simulink model "Octocopter2D"  (R2017b)
settings: Solver=VariableStepAuto  StartTime=0.0  StopTime=10  MaxStep=1e-3  RelTol=1e-3
undefined symbols (not defined in the file): Initial
libraries: simulink_extras x2
settings Model: Creator=jeremie  LastModifiedBy=jeremie

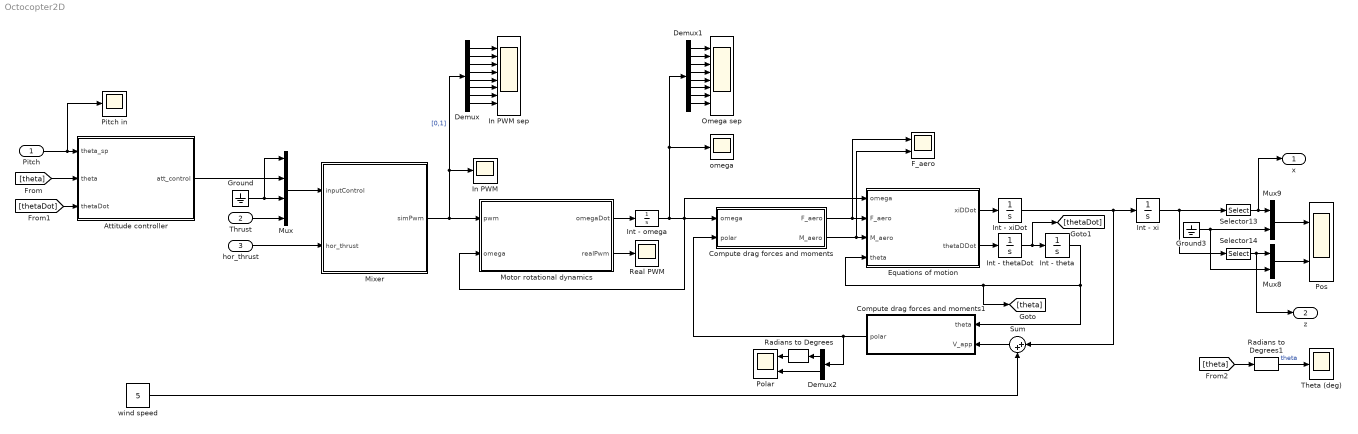
== system Octocopter2D ==
  Pitch : Inport
  Thrust : Inport  Port=2
  hor_thrust : Inport  Port=3
  Attitude controller : Subsystem
  Compute drag forces and moments : MATLAB Function  TreatAsAtomicUnit=on
  Compute drag forces and moments1 : MATLAB Function  TreatAsAtomicUnit=on
  Demux : Demux  Outputs=8
  Demux1 : Demux  Outputs=8
  Demux2 : Demux  Outputs=2
  Equations of motion : MATLAB Function  TreatAsAtomicUnit=on
  F_aero : Scope  NumInputPorts=2
  Ground : Ground
  Ground3 : Ground
  In PWM : Scope
  In PWM sep : Scope  NumInputPorts=8
  Int - omega : Integrator  InitialCondition=Initial.OMEGA
  Int - theta : Integrator
  Int - thetaDot : Integrator
  Int - xi : Integrator
  Int - xiDot : Integrator
  Mixer : MATLAB Function  TreatAsAtomicUnit=on
  Motor rotational dynamics : MATLAB Function  TreatAsAtomicUnit=on
  Mux : Mux
  Mux8 : Mux  Inputs=2
  Mux9 : Mux  Inputs=2
  Omega sep : Scope  NumInputPorts=8
  Pitch in : Scope
  Polar : Scope  NumInputPorts=2
  Pos : Scope  NumInputPorts=2
  Radians to Degrees : simulink_extras/Transformations/Radians to Degrees
  Radians to Degrees1 : simulink_extras/Transformations/Radians to Degrees
  Real PWM : Scope
  Selector13 : Selector  InputPortWidth=2  IndexOptions=Index vector (dialog)  Indices=1  OutputSizes=1
  Selector14 : Selector  InputPortWidth=2  IndexOptions=Index vector (dialog)  Indices=2  OutputSizes=1
  Sum : Sum  Inputs=|++
  Theta (deg) : Scope
  omega : Scope
  wind speed : Constant  Value=5
  x : Outport
  z : Outport  Port=2
  wires:
  Int - omega/1 -> Equations of motion/1(omega), Compute drag forces and moments/1(omega), Motor rotational dynamics/2(omega), omega/1, Demux1/1
  Compute drag forces and moments/1(F_aero) -> F_aero/1, Equations of motion/2(F_aero)
  Compute drag forces and moments/2(M_aero) -> F_aero/2, Equations of motion/3(M_aero)
  Motor rotational dynamics/1(omegaDot) -> Int - omega/1
  Motor rotational dynamics/2(realPwm) -> Real PWM/1
  Mixer/1(simPwm) -> Motor rotational dynamics/1(pwm), Demux/1, In PWM/1  "[0,1]"
  Mux/1 -> Mixer/1(inputControl)
  Ground/1 -> Mux/3, Mux/1
  Attitude controller/1(att_control) -> Mux/2
  Thrust/1 -> Mux/4
  Equations of motion/1(xiDDot) -> Int - xiDot/1
  Int - xiDot/1 -> Sum/1, Int - xi/1
  Equations of motion/2(thetaDDot) -> Int - thetaDot/1
  Int - thetaDot/1 -> [thetaDot], Int - theta/1
  Int - theta/1 -> [theta], Equations of motion/4(theta), Compute drag forces and moments1/1(theta)
  wind speed/1 -> Sum/2
  Sum/1 -> Compute drag forces and moments1/2(V_app)
  Compute drag forces and moments1/1(polar) -> Demux2/1, Compute drag forces and moments/2(polar)
  Ground3/1 -> Mux8/2, Mux9/2
  Selector14/1 -> z/1, Mux8/1
  Selector13/1 -> x/1, Mux9/1
  Mux8/1 -> Pos/2
  Mux9/1 -> Pos/1
  Int - xi/1 -> Selector14/1, Selector13/1
  Demux/1 -> In PWM sep/1
  Demux/2 -> In PWM sep/2
  Demux/3 -> In PWM sep/3
  Demux/4 -> In PWM sep/4
  Demux/5 -> In PWM sep/5
  Demux/6 -> In PWM sep/6
  Demux/7 -> In PWM sep/7
  Demux/8 -> In PWM sep/8
  Demux1/8 -> Omega sep/8
  Demux1/7 -> Omega sep/7
  Demux1/6 -> Omega sep/6
  Demux1/5 -> Omega sep/5
  Demux1/4 -> Omega sep/4
  Demux1/3 -> Omega sep/3
  Demux1/2 -> Omega sep/2
  Demux1/1 -> Omega sep/1
  Demux2/2 -> Polar/2
  Demux2/1 -> Radians to Degrees/1
  Radians to Degrees/1 -> Polar/1
  Radians to Degrees1/1 -> Theta (deg)/1  "theta"
  Pitch/1 -> Pitch in/1, Attitude controller/1(theta_sp)
  [theta] -> Attitude controller/2(theta)
  [thetaDot] -> Attitude controller/3(thetaDot)
  hor_thrust/1 -> Mixer/2(hor_thrust)
  [theta] -> Radians to Degrees1/1

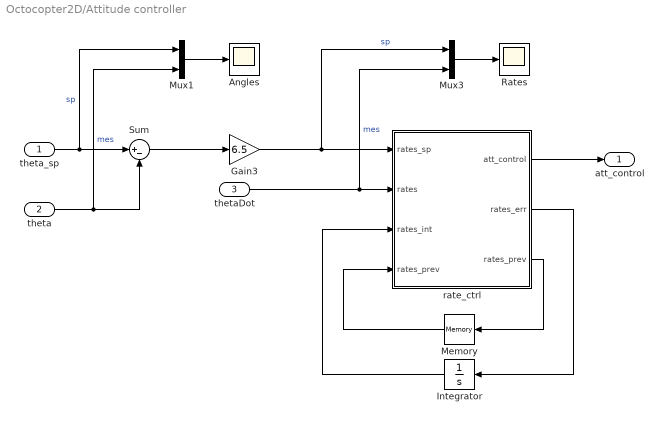
== system Octocopter2D/Attitude controller ==
  theta_sp : Inport
  theta : Inport  Port=2
  thetaDot : Inport  Port=3
  Angles : Scope
  Gain3 : Gain  Gain=6.5
  Integrator : Integrator
  Memory : Memory
  Mux1 : Mux  Inputs=2
  Mux3 : Mux  Inputs=2
  Rates : Scope
  Sum : Sum  Inputs=|+-
  rate_ctrl : MATLAB Function  TreatAsAtomicUnit=on  SystemSampleTime=0.002
  att_control : Outport
  wires:
  rate_ctrl/2(rates_err) -> Integrator/1
  rate_ctrl/3(rates_prev) -> Memory/1
  Integrator/1 -> rate_ctrl/3(rates_int)
  rate_ctrl/1(att_control) -> att_control/1
  Memory/1 -> rate_ctrl/4("rates_prev ")
  Mux3/1 -> Rates/1
  thetaDot/1 -> rate_ctrl/2(rates), Mux3/2  "mes"
  Gain3/1 -> rate_ctrl/1(rates_sp), Mux3/1  "sp"
  Sum/1 -> Gain3/1
  theta_sp/1 -> Mux1/1, Sum/1  "sp"
  theta/1 -> Mux1/2, Sum/2  "mes"
  Mux1/1 -> Angles/1

== matlab function Octocopter2D/Attitude controller/rate_ctrl ==
  data: rates_sp input size=1; rates input size=1; att_control output size=1; rates_err output; rates_prev output; rates_int input size=1; rates_prev input size=1
function [ att_control, rates_err, rates_prev ] = rate_ctrl(rates_sp, rates, rates_int, rates_prev)
rates_p = 0.15;
rates_i = 0.05;
rates_d = 0.003;
rate_ff = 0;

dt = 0.002;

% Angular rates error
rates_err = - rates_sp + rates;

% % Perform the integration using a first order method and do not propaate the result if out of range or invalid
% rates_int = rates_int +  rates_err * dt;

att_control = rates_p .* rates_err + rates_i .* rates_int + rates_d .* (rates_prev - rates) ./ dt + rate_ff .* rates_sp;

rates_prev = rates;

end

== matlab function Octocopter2D/Compute drag forces and moments ==
  data: omega input; polar input size=2; F_aero output; M_aero output; Uav parameter
function [F_aero, M_aero] = computeAero( omega, polar, Uav )
%#codegen

% Name variables
alpha    = -polar(1); % equations assume alpha measured the other way
U        = polar(2);
omegaBar = mean(omega);
rho      = Uav.RHO_AIR;
D_UAV    = Uav.D_UAV;
A_UAV    = Uav.A_UAV;
D_PROP   = Uav.D_PROP;
A_PROP   = Uav.A_PROP;
n        = Uav.N_ROTORS;

% Force coefficients
Cxb1 = -0.241*cos(alpha) + 0.036*cos(3*alpha) + 0.016*cos(7*alpha);
Cxb2 = -0.053*cos(alpha) - 0.008*cos(3*alpha);
Czb1 = -0.724*sin(alpha) + 0.080;
Czb2 = -0.222*sin(alpha) + 0.065;

% Moment coefficients
lambda = omegaBar*D_PROP / ( 2*U );
A1  =  0.116 * ( 1 - exp(-0.126*lambda) );
A2  = -0.041 * ( 1 - exp(-0.308*lambda) );
CM1 =  0.009*cos(alpha) + 0.003*cos(3*alpha) - 0.014*sin(2*alpha);
CM2 =  A1*cos(alpha) + A2*sin(2*alpha);

% Forces and moments
Fxb = 0.5*rho*U^2*Cxb1*A_UAV      + 0.5*rho*U*omegaBar*Cxb2*D_PROP*A_PROP*(n/4);
Fzb = 0.5*rho*U^2*Czb1*A_UAV      + 0.5*rho*U*omegaBar*Czb2*D_PROP*A_PROP*(n/4);
M   = 0.5*rho*U^2*CM1*A_UAV*D_UAV + 0.5*rho*U*omegaBar*CM2*D_PROP^2*A_PROP*(n/4);

% Output forces - NED
F_aero = [ Fxb; -Fzb ];
M_aero = M;

== matlab function Octocopter2D/Motor rotational dynamics ==
  data: pwm input; omegaDot output; omega input; realPwm output
function [omegaDot, realPwm]  = motorRotDynamics( pwm, omega)
%#codegen

realPwm = (1000 * pwm + 1000);
rotorTimeConst = 7.006512e-02;
omegaRef = zeros(8,1);
omegaRef = 0.84*(7.969173e-1 .* realPwm - 6.528579e2);

omegaDot = (omegaRef - omega) / rotorTimeConst;

== matlab function Octocopter2D/Equations of motion ==
  data: omega input; xiDDot output; F_aero input; M_aero input; theta input; thetaDDot output; Uav parameter
function [ xiDDot, thetaDDot ] = Octo2DModel( omega, F_aero, M_aero, theta, Uav )
%#codegen

% Name variables
m_UAV = Uav.M;
J_UAV = Uav.J;
C_T   = Uav.C_T;
D_UAV = Uav.D_UAV;
Fxb = F_aero(1);
Fzb = F_aero(2);
g = 9.80665;
zeta = Uav.ZETA;

% Forces and pitching moment in body frame
T   = -cos(zeta)*C_T*sum(omega.^2);
Txb = 2*sin(zeta)*C_T*(omega(3)^2 - omega(2)^2);

M = 2*cos(zeta)*D_UAV*C_T * ( ...
    omega(1)^2*sind(22.5) + omega(2)^2*cosd(22.5) - ...
    omega(3)^2*cosd(22.5) - omega(4)^2*sind(22.5) );

% Forces and pitching moment in world frame
xDDot = ( (T + Fzb)*sin(theta) + (Txb + Fxb)*cos(theta) ) / m_UAV;
zDDot = ( (T + Fzb)*cos(theta) + (Txb + Fxb)*sin(theta) + m_UAV*g ) / m_UAV;

xiDDot = [xDDot; zDDot];
thetaDDot = (M + M_aero) / J_UAV;

end

== matlab function Octocopter2D/Mixer ==
  data: inputControl input size=4; simPwm output size=8; hor_thrust input
function simPwm = mix( inputControl, hor_thrust )
%#codegen
    ROTOR_COUNT = 8;
    a = tand(22.5);
    rotors = struct( 'roll_scale',   {-0.095671,  0.095671, -0.230970, -0.095671,  0.095671,  0.230970,  0.230970, -0.230970}, ...
                     'pitch_scale',  { 0.230970, -0.230970,  0.095671, -0.230970,  0.230970, -0.095671,  0.095671, -0.095671}, ...
                     'yaw_scale',    {-2.500000, -2.500000,  2.500000,  2.500000,  2.500000,  2.500000, -2.500000, -2.500000}, ...
                     'thrust_scale', { 0.125000,  0.125000,  0.125000,  0.125000,  0.125000,  0.125000,  0.125000,  0.125000}, ...
                     'hor_thrust_scale', { a*1,  -a*1,  -1,  -a*1,  a*1,  1,  -1,  1});

%     roll   = constrain(inputControl(1), -1.0, 1.0);
%     pitch  = constrain(inputControl(2), -1.0, 1.0);
%     yaw    = constrain(inputControl(3), -1.0, 1.0);
%     thrust = constrain(inputControl(4), 0.0, 1.0);
%     min_out = 0.0;
%     max_out = 0.0;
%

    roll   = inputControl(1);
    pitch  = -inputControl(2);
    yaw    = -inputControl(3);
    thrust = inputControl(4);
    outputControl = zeros(ROTOR_COUNT,1);

    % /* perform initial mix pass yielding unbounded outputs, ignore yaw */
    for i = 1:ROTOR_COUNT
        out = pitch * rotors(i).pitch_scale + thrust + hor_thrust*rotors(i).hor_thrust_scale;%*rotors(i).thrust_scale;
%         out = roll * rotors(i).roll_scale ...
%                 + pitch * rotors(i).pitch_scale + thrust;
% 
%         % /* limit yaw if it causes outputs clipping */
%         if ( (out >= 0.0) && (out < (-yaw * rotors(i).yaw_scale) ) )
%             yaw = -out / rotors(i).yaw_scale;
%         end
% 
%         % /* calculate min and max output values */
%         if (out < min_out)
%             min_out = out;
%         end
% 
%         if (out > max_out)
%             max_out = out;
%         end

        outputControl(i) = out;
    end

%     % /* scale down roll/pitch controls if some outputs are negative, don't add yaw, keep total thrust */
%     if (min_out < 0.0)
%          scale_in = thrust / (thrust - min_out);
% 
%         % /* mix again with adjusted controls */
%         for i = 1:ROTOR_COUNT %(unsigned i = 0; i < _rotor_count; i++)
%             outputControl(i) = scale_in ...
%                          * (roll * rotors(i).roll_scale ...
%                         + pitch * rotors(i).pitch_scale) + thrust;
%         end
%     else
%         % /* roll/pitch mixed without limiting, add yaw control */
%         for i=1:ROTOR_COUNT %(unsigned i = 0; i < _rotor_count; i++)
%             outputControl(i) = outputControl(i) + yaw * rotors(i).yaw_scale;
%         end
%     end
% 
%     % /* scale down all outputs if some outputs are too large, reduce total thrust */
%     % scale_out;
% 
%     if (max_out > 1.0)
%         scale_out = 1.0 / max_out;
% 
%     else
%         scale_out = 1.0;
%     end
% 
%     % /* scale outputs to range _idle_speed..1, and do final limiting */
%     for i=1:ROTOR_COUNT %(unsigned i = 0; i < _rotor_count; i++)
%         outputControl(i) = constrain(outputControl(i) * scale_out, 0.0, 1.0); % added scale_out
%     end
    
    simPwm = [ outputControl(1); outputControl(3); outputControl(8); outputControl(4); outputControl(2); outputControl(6); outputControl(7); outputControl(5) ];
end

function y = constrain( x, x_min, x_max )
    y = max( min(x, x_max), x_min );
end

== matlab function Octocopter2D/Compute drag forces and moments1 ==
  data: theta input; V_app input; polar output
function polar   = computeSph( theta, V_app )
%#codegen

V_appBody = [ cos(theta), 0; 0, sin(theta) ] * V_app; % CHECK

% alpha = theta since wind is horizontal
polar = [theta; norm(V_appBody)];
